simulink model "s0506_polynomial_filter"  (R2019b)
settings: Solver=ode1  StartTime=0.0  StopTime=T_sim  FixedStep=dt_control  RelTol=1e-3
values from neighbouring files (symbols this model uses):
  dt_control = 2e-2    (= 0.02)    [m0310_init.m]    (also in m0312_init.m; m0314_init.m = 0.002; m0318_init.m = 0.002)
  PARAMS =     [s0310_main.mat]
undefined symbols (not defined in the file or in its folder): __PRM__SERIALIZED__DATA__, Continuous, Discrete, SubsystemReferenceBlock, Time
libraries: ctrlSharedLib x3
settings Model: Creator=paolo  LastModifiedBy=giaco
settings DebuggingCC: SFMachineParentedDataDiag=error  ArithmeticOperatorsInVariantConditions=warning
settings SFSimCC: CustomCodeUndefinedFunction=UseInterfaceOnly
settings CodeAppCC: StateflowObjectComments=on

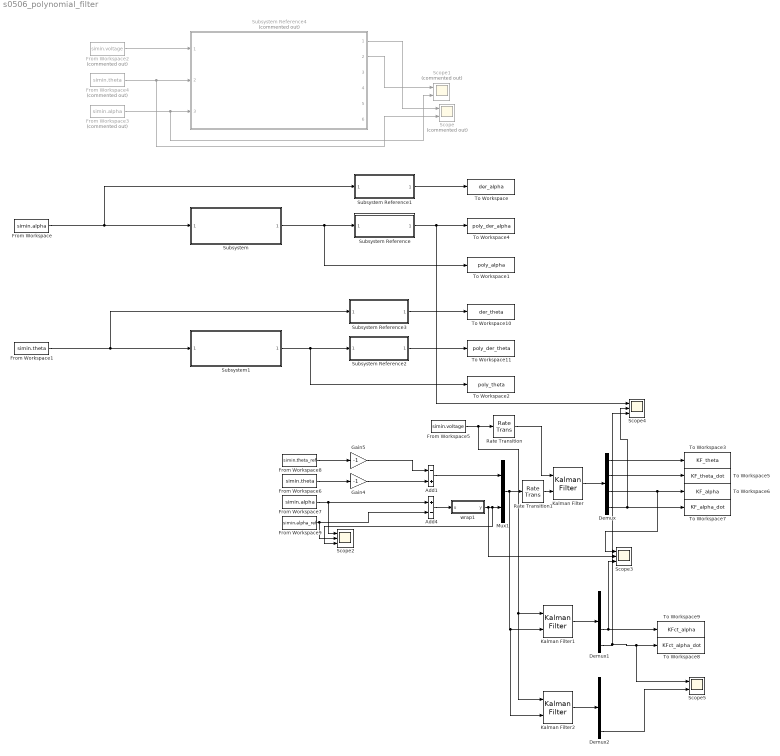
== system s0506_polynomial_filter ==
  Add1 : Sum  Inputs=-+
  Add4 : Sum  Inputs=+-
  Demux : Demux
  Demux1 : Demux
  Demux2 : Demux
  From Workspace : FromWorkspace  VariableName=simin.alpha  SampleTime=0
  From Workspace1 : FromWorkspace  VariableName=simin.theta  SampleTime=0
  From Workspace2 : FromWorkspace  Commented=on  VariableName=simin.voltage  SampleTime=0
  From Workspace3 : FromWorkspace  Commented=on  VariableName=simin.alpha  SampleTime=0
  From Workspace4 : FromWorkspace  Commented=on  VariableName=simin.theta  SampleTime=0
  From Workspace5 : FromWorkspace  VariableName=simin.voltage  SampleTime=0
  From Workspace6 : FromWorkspace  VariableName=simin.theta  SampleTime=0
  From Workspace7 : FromWorkspace  VariableName=simin.alpha  SampleTime=0
  From Workspace8 : FromWorkspace  VariableName=simin.theta_ref  SampleTime=0
  From Workspace9 : FromWorkspace  VariableName=simin.alpha_ref  SampleTime=0
  Gain4 : Gain  Gain=-1
  Gain5 : Gain  Gain=-1
  Kalman Filter : ctrlSharedLib/Kalman Filter  TimeDomain=Discrete-Time  UseCurrentEstimator=on  ModelSource=Individual A, B, C, D matrices  ModelSourceVariable=ss(0.95,1,1,0,1)  A=PARAMS.A_pi_DT  B=PARAMS.B_pi_DT  C=[1 0 0 0; 0 0 1 0]  D=[0; 0]  NumberOfStates=1  NumberOfInputs=1  NumberOfOutputs=1  InitialEstimateSource=Dialog  X0=[PARAMS.th_0, PARAMS.th_dot_0, 0, PARAMS.al_dot_0]  P0=10  UseK=off  UseGH=off  NumberOfProcessNoiseInputs=1  G=1  TimeInvariantG=on  H=0  TimeInvariantH=on  Q=diag([1, 1e8, 1, 1e8]);  TimeInvariantQ=on  R=diag([1e5, 1e5]);  TimeInvariantR=on  N=0  TimeInvariantN=on  AddInputPort=on  AddEnablePort=off  OutputEstimatedY=off  OutputP=off  Ts=dt_control
      settings: SourceProductBaseCode=CT
  Kalman Filter1 : ctrlSharedLib/Kalman Filter  TimeDomain=Continuous-Time  UseCurrentEstimator=on  ModelSource=Individual A, B, C, D matrices  ModelSourceVariable=ss(0.95,1,1,0,1)  A=PARAMS.A_pi_CT  B=PARAMS.B_pi_CT  C=[1 0 0 0; 0 0 1 0]  D=[0; 0]  NumberOfStates=1  NumberOfInputs=1  NumberOfOutputs=1  InitialEstimateSource=Dialog  X0=[PARAMS.th_0, PARAMS.th_dot_0, 0, PARAMS.al_dot_0]  P0=10  UseK=off  UseGH=off  NumberOfProcessNoiseInputs=1  G=1  TimeInvariantG=on  H=0  TimeInvariantH=on  Q=diag([1, 1e8, 1, 1e8]);  TimeInvariantQ=on  R=diag([1, 1]);  TimeInvariantR=on  N=0  TimeInvariantN=on  AddInputPort=on  AddEnablePort=off  OutputEstimatedY=off  OutputP=off  Ts=dt_control
      settings: SourceProductBaseCode=CT
  Kalman Filter2 : ctrlSharedLib/Kalman Filter  TimeDomain=Continuous-Time  UseCurrentEstimator=on  ModelSource=Individual A, B, C, D matrices  ModelSourceVariable=ss(0.95,1,1,0,1)  A=PARAMS.A_pi_CT  B=PARAMS.B_pi_CT  C=[1 0 0 0; 0 0 1 0]  D=[0; 0]  NumberOfStates=1  NumberOfInputs=1  NumberOfOutputs=1  InitialEstimateSource=Dialog  X0=[PARAMS.th_0, PARAMS.th_dot_0, 0, PARAMS.al_dot_0]  P0=10  UseK=off  UseGH=off  NumberOfProcessNoiseInputs=1  G=1  TimeInvariantG=on  H=0  TimeInvariantH=on  Q=diag([1, 1e8, 1, 1e8]);  TimeInvariantQ=on  R=diag([100, 100]);  TimeInvariantR=on  N=0  TimeInvariantN=on  AddInputPort=on  AddEnablePort=off  OutputEstimatedY=off  OutputP=off  Ts=dt_control
      settings: SourceProductBaseCode=CT
  Mux1 : Mux  Inputs=2
  Rate Transition : RateTransition  OutPortSampleTime=dt_control
  Rate Transition1 : RateTransition  OutPortSampleTime=dt_control
  Scope : Scope  Commented=on  NumInputPorts=2
  Scope1 : Scope  Commented=on  NumInputPorts=2
  Scope2 : Scope  NumInputPorts=3
  Scope3 : Scope  NumInputPorts=3
  Scope4 : Scope  NumInputPorts=3
  Scope5 : Scope  NumInputPorts=2
  Subsystem : Subsystem  ReferencedSubsystem=Polynomial_Filter
  Subsystem Reference{,1..3} (4 alike) : Subsystem  BlockKeywords=__PRM__SERIALIZED__DATA__:SubsystemReferenceBlock  ReferencedSubsystem=Filtered_Derivative  num=num_der_filter  den=den_der_filter
  Subsystem Reference4 : Subsystem  Commented=on  BlockKeywords=__PRM__SERIALIZED__DATA__:SubsystemReferenceBlock  ReferencedSubsystem=s0606_SIL_observer  th_0=PARAMS.th_0  al_0=PARAMS.al_0  th_dot_0=PARAMS.th_dot_0  al_dot_0=PARAMS.al_dot_0
  Subsystem1 : Subsystem  ReferencedSubsystem=Polynomial_Filter
  To Workspace : ToWorkspace  VariableName=der_alpha  SaveFormat=Timeseries  SampleTime=-1
  To Workspace1 : ToWorkspace  VariableName=poly_alpha  SaveFormat=Timeseries  SampleTime=-1
  To Workspace10 : ToWorkspace  VariableName=der_theta  SaveFormat=Timeseries  SampleTime=-1
  To Workspace11 : ToWorkspace  VariableName=poly_der_theta  SaveFormat=Timeseries  SampleTime=-1
  To Workspace2 : ToWorkspace  VariableName=poly_theta  SaveFormat=Timeseries  SampleTime=-1
  To Workspace3 : ToWorkspace  VariableName=KF_theta  SaveFormat=Timeseries  SampleTime=-1
  To Workspace4 : ToWorkspace  VariableName=poly_der_alpha  SaveFormat=Timeseries  SampleTime=-1
  To Workspace5 : ToWorkspace  VariableName=KF_theta_dot  SaveFormat=Timeseries  SampleTime=-1
  To Workspace6 : ToWorkspace  VariableName=KF_alpha  SaveFormat=Timeseries  SampleTime=-1
  To Workspace7 : ToWorkspace  VariableName=KF_alpha_dot  SaveFormat=Timeseries  SampleTime=-1
  To Workspace8 : ToWorkspace  VariableName=KFct_alpha_dot  SaveFormat=Timeseries  SampleTime=-1
  To Workspace9 : ToWorkspace  VariableName=KFct_alpha  SaveFormat=Timeseries  SampleTime=-1
  wrap1 : MATLAB Function  TreatAsAtomicUnit=on
  wires:
  From Workspace/1 -> Subsystem/1, Subsystem Reference1/1
  From Workspace1/1 -> Subsystem1/1, Subsystem Reference3/1
  Subsystem Reference1/1 -> To Workspace/1
  Subsystem Reference/1 -> Scope4/1, To Workspace4/1
  Subsystem Reference3/1 -> To Workspace10/1
  Subsystem Reference2/1 -> To Workspace11/1
  Subsystem/1 -> To Workspace1/1, Subsystem Reference/1
  Subsystem1/1 -> To Workspace2/1, Subsystem Reference2/1
  From Workspace2/1 -> Subsystem Reference4/1
  From Workspace3/1 -> Scope1/2, Subsystem Reference4/3
  From Workspace4/1 -> Scope/2, Subsystem Reference4/2
  Subsystem Reference4/1 -> Scope/1
  Subsystem Reference4/2 -> Scope1/1
  From Workspace8/1 -> Gain5/1
  Add1/1 -> Mux1/1
  Gain4/1 -> Add1/2
  From Workspace7/1 -> Scope2/1, Add4/1
  Add4/1 -> wrap1/1(u)
  wrap1/1(y) -> Scope3/2, Scope2/3, Mux1/2
  From Workspace9/1 -> Scope2/2, Add4/2
  From Workspace6/1 -> Gain4/1
  Gain5/1 -> Add1/1
  From Workspace5/1 -> Kalman Filter2/1, Kalman Filter1/1, Rate Transition/1
  Rate Transition/1 -> Kalman Filter/1
  Kalman Filter/1 -> Demux/1
  Demux/3 -> Scope3/1, To Workspace6/1
  Demux/4 -> Scope4/2, To Workspace7/1
  Demux/2 -> To Workspace5/1
  Demux/1 -> To Workspace3/1
  Rate Transition1/1 -> Kalman Filter/2
  Mux1/1 -> Kalman Filter2/2, Kalman Filter1/2, Rate Transition1/1
  Kalman Filter1/1 -> Demux1/1
  Demux1/3 -> Scope3/3, To Workspace9/1
  Demux1/4 -> Scope5/1, To Workspace8/1, Scope4/3
  Kalman Filter2/1 -> Demux2/1
  Demux2/4 -> Scope5/2

== matlab function s0506_polynomial_filter/wrap1 ==
  data: u input; y output
function y = wrap(u)
stop_condition = false;
y = u;
while ~stop_condition
    if y > pi
        y = y - 2*pi;
    elseif y < -pi
        y = y + 2*pi;
    else
        stop_condition = true;
    end
end
